simulink model "SF044A_HowDetn"  (R2013b)
settings: Solver=FixedStepDiscrete  SolverMode=SingleTasking  StartTime=0.0  StopTime=1  FixedStep=0.002  RelTol=1e-3
values from neighbouring files (symbols this model uses):
  ABSLTHIFRQTQHILIM_HWNWTMTR_F32 = DataDict.Constant    [SF044A_HowDetn_DataDict.m]
  ABSLTHIFRQTQLOLIM_HWNWTMTR_F32 = DataDict.Constant    [SF044A_HowDetn_DataDict.m]
  ARCHGLBPRM_2MILLISEC_SEC_F32 = DataDict.Constant    [SF044A_HowDetn_DataDict.m]
  HOWDETNESTIMNLIM_ULS_F32 = DataDict.Constant    [SF044A_HowDetn_DataDict.m]
  HOWDETNESTIMNTHD_ULS_F32 = DataDict.Constant    [SF044A_HowDetn_DataDict.m]
  HowDetnHiFrqGainY = DataDict.Calibration    [SF044A_HowDetn_DataDict.m]
  HowDetnMinVehSpd = DataDict.Calibration    [SF044A_HowDetn_DataDict.m]
  HowDetnOffThd = DataDict.Calibration    [SF044A_HowDetn_DataDict.m]
  HowDetnOffTi = DataDict.Calibration    [SF044A_HowDetn_DataDict.m]
  HowDetnPercOfPrevHowEstim = DataDict.Calibration    [SF044A_HowDetn_DataDict.m]
  HowDetnSlewRate = DataDict.Calibration    [SF044A_HowDetn_DataDict.m]
  HowDetnVehSpd = DataDict.Calibration    [SF044A_HowDetn_DataDict.m]
  HUNDREDMICROSECTOMILLISEC_ULS_F32 = DataDict.Constant    [SF044A_HowDetn_DataDict.m]
  MILLISECTOSEC_ULS_F32 = DataDict.Constant    [SF044A_HowDetn_DataDict.m]
libraries: Fil x14, FloatToFixd x6, NxtrLim x5, FixdToFloat x4, BilnrIntrpnMplX x2, NxtrAbslt x2, simulink x2, LnrIntrpn x1, LnrIntrpnDyn x1
(part 2 of 2)

== system SF044A_HowDetn/HowDetn/HowDetnPer1/Calculate HOW Estimate/Low-Frequency Lookup Table ==
  VehSpd : Inport
  AbsLoFrqTq : Inport  Port=2
  BilnrIntrpnWithRound_s16_u16MplXs16MplY : BilnrIntrpnMplX/BilnrIntrpnWithRound_s16_u16MplXs16MplY  MplXTbl=HowDetnLoFrqRateX  MplYTbl=HowDetnLoFrqRateY  BilnrSelnTbl=HowDetnVehSpd
      settings: AttributesFormatString=Bilnr ( u16MplX , s16MplY )
  CopyRight2 : Subsystem  Description=|  mask(Copyright Information){none=on}
      | Copyright info block.                                               
      |                                                                     
      | Place copyright information at the top of every subsystem in design.
      mask prompts: none "No parameters"
      mask help: Place copyright information at the top of every subsystem in design.
      mask Display:
      | NxtrConf = 'Nexteer Confidential';
      | 
      | sys = bdroot; %handle for the current model ("system")
      | first = get_param(sys,'Created');
      | first = first(end-3:end);  %year is last four digits
      | 
      | last = get_param(sys,'LastModifiedDate');
      | if isempty(last)
      |     last = datestr(now,'yyyy');
      | else
      |     last = last(end-3:end);
      | end
      | 
      | if strcmp(first,last)
      |     fprintf('%s -- Copyright %s Nexteer',NxtrConf,first)
      | else
      |     fprintf('%s -- %s%s- %s Nexteer',NxtrConf,char(169),first,last)
      | end
  FixdToFloat_f32_s16 : FixdToFloat/FixdToFloat_f32_s16  Param1=8
  FloatToFixd_u16_f1 : FloatToFixd/FloatToFixd_u16_f32  Param1=8
  FloatToFixd_u16_f32 : FloatToFixd/FloatToFixd_u16_f32  Param1=7
  LoFrqRateY : Outport
  wires:
  FloatToFixd_u16_f32/1 -> BilnrIntrpnWithRound_s16_u16MplXs16MplY/2
  BilnrIntrpnWithRound_s16_u16MplXs16MplY/1 -> FixdToFloat_f32_s16/1
  FloatToFixd_u16_f1/1 -> BilnrIntrpnWithRound_s16_u16MplXs16MplY/1
  VehSpd/1 -> FloatToFixd_u16_f32/1
  AbsLoFrqTq/1 -> FloatToFixd_u16_f1/1
  FixdToFloat_f32_s16/1 -> LoFrqRateY/1

== system SF044A_HowDetn/HowDetn/HowDetnPer1/Calculate HOW Estimate/default ==
  Action Port : ActionPort  ActionType=else
  Constant : Constant  RequirementInfo={} %GIDa_67017ff9_6322_4976_b2c8_c00694960ef8  Value=HOWDETNESTIMNTHD_ULS_F32  OutDataTypeStr=single
  CopyRight2 : Subsystem  Description=|  mask(Copyright Information){none=on}
      | Copyright info block.                                               
      |                                                                     
      | Place copyright information at the top of every subsystem in design.
      mask prompts: none "No parameters"
      mask help: Place copyright information at the top of every subsystem in design.
      mask Display:
      | NxtrConf = 'Nexteer Confidential';
      | 
      | sys = bdroot; %handle for the current model ("system")
      | first = get_param(sys,'Created');
      | first = first(end-3:end);  %year is last four digits
      | 
      | last = get_param(sys,'LastModifiedDate');
      | if isempty(last)
      |     last = datestr(now,'yyyy');
      | else
      |     last = last(end-3:end);
      | end
      | 
      | if strcmp(first,last)
      |     fprintf('%s -- Copyright %s Nexteer',NxtrConf,first)
      | else
      |     fprintf('%s -- %s%s- %s Nexteer',NxtrConf,char(169),first,last)
      | end
  Out : Outport
  wires:
  Constant/1 -> Out/1

== system SF044A_HowDetn/HowDetn/HowDetnPer1/Determine HOW Flag/CopyRight2 ==

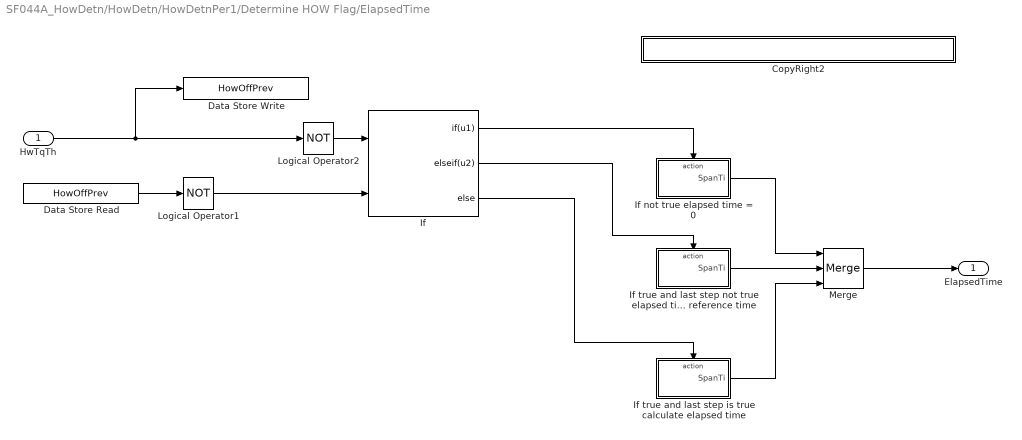
== system SF044A_HowDetn/HowDetn/HowDetnPer1/Determine HOW Flag/ElapsedTime ==
  HwTqTh : Inport
  CopyRight2 : Subsystem  Description=|  mask(Copyright Information){none=on}
      | Copyright info block.                                               
      |                                                                     
      | Place copyright information at the top of every subsystem in design.
      mask prompts: none "No parameters"
      mask help: Place copyright information at the top of every subsystem in design.
      mask Display:
      | NxtrConf = 'Nexteer Confidential';
      | 
      | sys = bdroot; %handle for the current model ("system")
      | first = get_param(sys,'Created');
      | first = first(end-3:end);  %year is last four digits
      | 
      | last = get_param(sys,'LastModifiedDate');
      | if isempty(last)
      |     last = datestr(now,'yyyy');
      | else
      |     last = last(end-3:end);
      | end
      | 
      | if strcmp(first,last)
      |     fprintf('%s -- Copyright %s Nexteer',NxtrConf,first)
      | else
      |     fprintf('%s -- %s%s- %s Nexteer',NxtrConf,char(169),first,last)
      | end
  Data Store Read : DataStoreRead  Priority=0  DataStoreName=HowOffPrev
      settings: AttributesFormatString=Priority: %<Priority>
  Data Store Write : DataStoreWrite  Priority=1  DataStoreName=HowOffPrev
      settings: AttributesFormatString=Priority: %<Priority>
  If : If  NumInputs=2  IfExpression=u1  ElseIfExpressions=u2
  If not true elapsed time = 0 : Subsystem  TreatAsAtomicUnit=on
  "If true and last step is true calculate elapsed time " : Subsystem  TreatAsAtomicUnit=on
  "If true and last step not true elapsed time = 0 get reference time " : Subsystem  TreatAsAtomicUnit=on
  Logical Operator1 : Logic  Operator=NOT  AllPortsSameDT=off  OutDataTypeStr=boolean
  Logical Operator2 : Logic  Operator=NOT  AllPortsSameDT=off  OutDataTypeStr=boolean
  Merge : Merge  Inputs=3
  ElapsedTime : Outport
  wires:
  If/1 -> If not true elapsed time = 0/Action
  If/2 -> "If true and last step not true elapsed time = 0 get reference time "/Action
  If/3 -> "If true and last step is true calculate elapsed time "/Action
  If not true elapsed time = 0/1(SpanTi) -> Merge/1
  "If true and last step not true elapsed time = 0 get reference time "/1("SpanTi ") -> Merge/2
  "If true and last step is true calculate elapsed time "/1(SpanTi) -> Merge/3
  Merge/1 -> ElapsedTime/1
  HwTqTh/1 -> Logical Operator2/1, Data Store Write/1
  Data Store Read/1 -> Logical Operator1/1
  Logical Operator2/1 -> If/1
  Logical Operator1/1 -> If/2

== system SF044A_HowDetn/HowDetn/HowDetnPer1/Determine HOW Flag/HandsOffDetn ==
  Action Port : ActionPort  ActionType=then
  CopyRight2 : Subsystem  Description=|  mask(Copyright Information){none=on}
      | Copyright info block.                                               
      |                                                                     
      | Place copyright information at the top of every subsystem in design.
      mask prompts: none "No parameters"
      mask help: Place copyright information at the top of every subsystem in design.
      mask Display:
      | NxtrConf = 'Nexteer Confidential';
      | 
      | sys = bdroot; %handle for the current model ("system")
      | first = get_param(sys,'Created');
      | first = first(end-3:end);  %year is last four digits
      | 
      | last = get_param(sys,'LastModifiedDate');
      | if isempty(last)
      |     last = datestr(now,'yyyy');
      | else
      |     last = last(end-3:end);
      | end
      | 
      | if strcmp(first,last)
      |     fprintf('%s -- Copyright %s Nexteer',NxtrConf,first)
      | else
      |     fprintf('%s -- %s%s- %s Nexteer',NxtrConf,char(169),first,last)
      | end
  Hands Off Wheel : Constant  RequirementInfo={} %GIDa_d4e6488b_e252_4824_9c02_dd6a1a50822f  Value=false  OutDataTypeStr=boolean
  HowDetnFlg : Outport
  wires:
  Hands Off Wheel/1 -> HowDetnFlg/1

== system SF044A_HowDetn/HowDetn/HowDetnPer1/Determine HOW Flag/HandsOnDetn ==
  Action Port : ActionPort  ActionType=else
  CopyRight2 : Subsystem  Description=|  mask(Copyright Information){none=on}
      | Copyright info block.                                               
      |                                                                     
      | Place copyright information at the top of every subsystem in design.
      mask prompts: none "No parameters"
      mask help: Place copyright information at the top of every subsystem in design.
      mask Display:
      | NxtrConf = 'Nexteer Confidential';
      | 
      | sys = bdroot; %handle for the current model ("system")
      | first = get_param(sys,'Created');
      | first = first(end-3:end);  %year is last four digits
      | 
      | last = get_param(sys,'LastModifiedDate');
      | if isempty(last)
      |     last = datestr(now,'yyyy');
      | else
      |     last = last(end-3:end);
      | end
      | 
      | if strcmp(first,last)
      |     fprintf('%s -- Copyright %s Nexteer',NxtrConf,first)
      | else
      |     fprintf('%s -- %s%s- %s Nexteer',NxtrConf,char(169),first,last)
      | end
  Hands On Wheel : Constant  RequirementInfo={} %GIDa_8392a09a_cc4f_428e_9a0f_d9eb35861263  Value=true  OutDataTypeStr=boolean
  HowDetnFlg : Outport
  wires:
  Hands On Wheel/1 -> HowDetnFlg/1

== system SF044A_HowDetn/HowDetn/HowDetnPer1/Determine HOW State/CopyRight2 ==

== system SF044A_HowDetn/HowDetn/HowDetnPer1/Determine HOW State/HOW State Look up Table ==
  HowEstimFil : Inport
  CopyRight2 : Subsystem  Description=|  mask(Copyright Information){none=on}
      | Copyright info block.                                               
      |                                                                     
      | Place copyright information at the top of every subsystem in design.
      mask prompts: none "No parameters"
      mask help: Place copyright information at the top of every subsystem in design.
      mask Display:
      | NxtrConf = 'Nexteer Confidential';
      | 
      | sys = bdroot; %handle for the current model ("system")
      | first = get_param(sys,'Created');
      | first = first(end-3:end);  %year is last four digits
      | 
      | last = get_param(sys,'LastModifiedDate');
      | if isempty(last)
      |     last = datestr(now,'yyyy');
      | else
      |     last = last(end-3:end);
      | end
      | 
      | if strcmp(first,last)
      |     fprintf('%s -- Copyright %s Nexteer',NxtrConf,first)
      | else
      |     fprintf('%s -- %s%s- %s Nexteer',NxtrConf,char(169),first,last)
      | end
  Data Type Conversion : DataTypeConversion  OutDataTypeStr=int8
  FloatToFixd_u16_f1 : FloatToFixd/FloatToFixd_u16_f32  Param1=8
  LnrIntrpn_s16_u16VariXs16VariY : LnrIntrpn/LnrIntrpn_s16_u16VariXs16VariY  RequirementInfo={} %GIDa_1ceff8d9_cb44_435a_8fb8_bb742ada6bbe  XTbl=HowDetnStThdX  YTbl=HOWSTY_CNT_S15P0
      settings: AttributesFormatString=Lnr ( u16VariX , s16VariY )
  HowDetnSt : Outport
  wires:
  HowEstimFil/1 -> FloatToFixd_u16_f1/1
  FloatToFixd_u16_f1/1 -> LnrIntrpn_s16_u16VariXs16VariY/1
  LnrIntrpn_s16_u16VariXs16VariY/1 -> Data Type Conversion/1
  Data Type Conversion/1 -> HowDetnSt/1

== system SF044A_HowDetn/HowDetn/HowDetnPer1/Determine HOW State/Pass ==
  Input : Inport
  Action Port : ActionPort  ActionType=then
  CopyRight2 : Subsystem  Description=|  mask(Copyright Information){none=on}
      | Copyright info block.                                               
      |                                                                     
      | Place copyright information at the top of every subsystem in design.
      mask prompts: none "No parameters"
      mask help: Place copyright information at the top of every subsystem in design.
      mask Display:
      | NxtrConf = 'Nexteer Confidential';
      | 
      | sys = bdroot; %handle for the current model ("system")
      | first = get_param(sys,'Created');
      | first = first(end-3:end);  %year is last four digits
      | 
      | last = get_param(sys,'LastModifiedDate');
      | if isempty(last)
      |     last = datestr(now,'yyyy');
      | else
      |     last = last(end-3:end);
      | end
      | 
      | if strcmp(first,last)
      |     fprintf('%s -- Copyright %s Nexteer',NxtrConf,first)
      | else
      |     fprintf('%s -- %s%s- %s Nexteer',NxtrConf,char(169),first,last)
      | end
  HowDetnSt : Outport
  wires:
  Input/1 -> HowDetnSt/1

== system SF044A_HowDetn/HowDetn/HowDetnPer1/Determine HOW State/Zero ==
  Action Port : ActionPort  ActionType=else
  Constant : Constant  Value=0  OutDataTypeStr=int8
      settings: AttributesFormatString=%<OutDataTypeStr>
  CopyRight2 : Subsystem  Description=|  mask(Copyright Information){none=on}
      | Copyright info block.                                               
      |                                                                     
      | Place copyright information at the top of every subsystem in design.
      mask prompts: none "No parameters"
      mask help: Place copyright information at the top of every subsystem in design.
      mask Display:
      | NxtrConf = 'Nexteer Confidential';
      | 
      | sys = bdroot; %handle for the current model ("system")
      | first = get_param(sys,'Created');
      | first = first(end-3:end);  %year is last four digits
      | 
      | last = get_param(sys,'LastModifiedDate');
      | if isempty(last)
      |     last = datestr(now,'yyyy');
      | else
      |     last = last(end-3:end);
      | end
      | 
      | if strcmp(first,last)
      |     fprintf('%s -- Copyright %s Nexteer',NxtrConf,first)
      | else
      |     fprintf('%s -- %s%s- %s Nexteer',NxtrConf,char(169),first,last)
      | end
  HowDetnSt : Outport
  wires:
  Constant/1 -> HowDetnSt/1

== system SF044A_HowDetn/HowDetn/HowDetnPer1/Filter HwTq/CopyRight2 ==

== system SF044A_HowDetn/HowDetn/HowDetnPer1/Calculate HOW Estimate/CalcEstimn/CopyRight2 ==

== system SF044A_HowDetn/HowDetn/HowDetnPer1/Calculate HOW Estimate/High-Frequency Lookup Table/CopyRight2 ==

== system SF044A_HowDetn/HowDetn/HowDetnPer1/Calculate HOW Estimate/Low-Frequency Lookup Table/CopyRight2 ==

== system SF044A_HowDetn/HowDetn/HowDetnPer1/Calculate HOW Estimate/default/CopyRight2 ==

== system SF044A_HowDetn/HowDetn/HowDetnPer1/Determine HOW Flag/ElapsedTime/CopyRight2 ==

== system SF044A_HowDetn/HowDetn/HowDetnPer1/Determine HOW Flag/ElapsedTime/If not true elapsed time = 0 ==
  Action Port : ActionPort  ActionType=then
  Constant : Constant  Value=0  OutDataTypeStr=single
  CopyRight2 : Subsystem  Description=|  mask(Copyright Information){none=on}
      | Copyright info block.                                               
      |                                                                     
      | Place copyright information at the top of every subsystem in design.
      mask prompts: none "No parameters"
      mask help: Place copyright information at the top of every subsystem in design.
      mask Display:
      | NxtrConf = 'Nexteer Confidential';
      | 
      | sys = bdroot; %handle for the current model ("system")
      | first = get_param(sys,'Created');
      | first = first(end-3:end);  %year is last four digits
      | 
      | last = get_param(sys,'LastModifiedDate');
      | if isempty(last)
      |     last = datestr(now,'yyyy');
      | else
      |     last = last(end-3:end);
      | end
      | 
      | if strcmp(first,last)
      |     fprintf('%s -- Copyright %s Nexteer',NxtrConf,first)
      | else
      |     fprintf('%s -- %s%s- %s Nexteer',NxtrConf,char(169),first,last)
      | end
  SpanTi : Outport
  wires:
  Constant/1 -> SpanTi/1

== system SF044A_HowDetn/HowDetn/HowDetnPer1/Determine HOW Flag/ElapsedTime/If true and last step is true calculate elapsed time  ==
  Action Port : ActionPort  ActionType=else
  Constant1 : Constant  Value=HUNDREDMICROSECTOMILLISEC_ULS_F32
  CopyRight2 : Subsystem  Description=|  mask(Copyright Information){none=on}
      | Copyright info block.                                               
      |                                                                     
      | Place copyright information at the top of every subsystem in design.
      mask prompts: none "No parameters"
      mask help: Place copyright information at the top of every subsystem in design.
      mask Display:
      | NxtrConf = 'Nexteer Confidential';
      | 
      | sys = bdroot; %handle for the current model ("system")
      | first = get_param(sys,'Created');
      | first = first(end-3:end);  %year is last four digits
      | 
      | last = get_param(sys,'LastModifiedDate');
      | if isempty(last)
      |     last = datestr(now,'yyyy');
      | else
      |     last = last(end-3:end);
      | end
      | 
      | if strcmp(first,last)
      |     fprintf('%s -- Copyright %s Nexteer',NxtrConf,first)
      | else
      |     fprintf('%s -- %s%s- %s Nexteer',NxtrConf,char(169),first,last)
      | end
  Data Store Read : DataStoreRead  DataStoreName=RefTiHowOff
  Divide : Product  Inputs=**
  FixdToFloat_f32_u32 : FixdToFloat/FixdToFloat_f32_u32  Param1=0
  GetTiSpan100MicroSec32bit : Subsystem  mask(Timer_GTS){}
      mask help: Used to get the time span between start and current time.
  SpanTi : Outport
  wires:
  Divide/1 -> SpanTi/1
  GetTiSpan100MicroSec32bit/1(TiSpan) -> FixdToFloat_f32_u32/1
  Data Store Read/1 -> GetTiSpan100MicroSec32bit/1(RefTmr)
  FixdToFloat_f32_u32/1 -> Divide/1
  Constant1/1 -> Divide/2

== system SF044A_HowDetn/HowDetn/HowDetnPer1/Determine HOW Flag/ElapsedTime/If true and last step not true elapsed time = 0 get reference time  ==
  Action Port : ActionPort  ActionType=elseif
  Constant : Constant  Value=0  OutDataTypeStr=single
  CopyRight2 : Subsystem  Description=|  mask(Copyright Information){none=on}
      | Copyright info block.                                               
      |                                                                     
      | Place copyright information at the top of every subsystem in design.
      mask prompts: none "No parameters"
      mask help: Place copyright information at the top of every subsystem in design.
      mask Display:
      | NxtrConf = 'Nexteer Confidential';
      | 
      | sys = bdroot; %handle for the current model ("system")
      | first = get_param(sys,'Created');
      | first = first(end-3:end);  %year is last four digits
      | 
      | last = get_param(sys,'LastModifiedDate');
      | if isempty(last)
      |     last = datestr(now,'yyyy');
      | else
      |     last = last(end-3:end);
      | end
      | 
      | if strcmp(first,last)
      |     fprintf('%s -- Copyright %s Nexteer',NxtrConf,first)
      | else
      |     fprintf('%s -- %s%s- %s Nexteer',NxtrConf,char(169),first,last)
      | end
  Data Store Write : DataStoreWrite  DataStoreName=RefTiHowOff
  GetRefTmr100MicroSec32bit1 : Subsystem  mask(Timer_GRF){}
      mask help: Used to get the reference time in a model.
  "SpanTi " : Outport
  wires:
  Constant/1 -> "SpanTi "/1
  GetRefTmr100MicroSec32bit1/1(RefTmr) -> Data Store Write/1

== system SF044A_HowDetn/HowDetn/HowDetnPer1/Determine HOW Flag/HandsOffDetn/CopyRight2 ==

== system SF044A_HowDetn/HowDetn/HowDetnPer1/Determine HOW Flag/HandsOnDetn/CopyRight2 ==

== system SF044A_HowDetn/HowDetn/HowDetnPer1/Determine HOW State/HOW State Look up Table/CopyRight2 ==

== system SF044A_HowDetn/HowDetn/HowDetnPer1/Determine HOW State/Pass/CopyRight2 ==

== system SF044A_HowDetn/HowDetn/HowDetnPer1/Determine HOW State/Zero/CopyRight2 ==

== system SF044A_HowDetn/HowDetn/HowDetnPer1/Determine HOW Flag/ElapsedTime/If not true elapsed time = 0/CopyRight2 ==

== system SF044A_HowDetn/HowDetn/HowDetnPer1/Determine HOW Flag/ElapsedTime/If true and last step is true calculate elapsed time /CopyRight2 ==

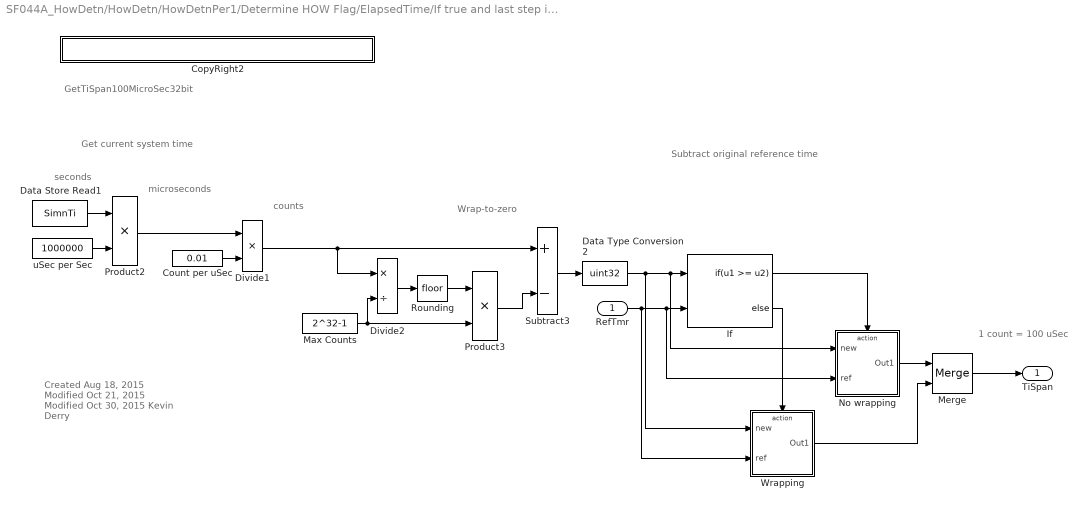
== system SF044A_HowDetn/HowDetn/HowDetnPer1/Determine HOW Flag/ElapsedTime/If true and last step is true calculate elapsed time /GetTiSpan100MicroSec32bit ==
  note: Subtract original reference time
  note: seconds
  note: microseconds
  note: counts
  note: Wrap-to-zero
  note: 1 count = 100 uSec
  note: Get current system time
  note: GetTiSpan100MicroSec32bit
  note: Created Aug 18, 2015
      | Modified Oct 21, 2015
      | Modified Oct 30, 2015
      | Kevin Derry
  RefTmr : Inport
  CopyRight2 : Subsystem  Description=|  mask(Copyright Information){none=on}
      | Copyright info block.                                               
      |                                                                     
      | Place copyright information at the top of every subsystem in design.
      mask prompts: none "No parameters"
      mask help: Place copyright information at the top of every subsystem in design.
      mask Display:
      | NxtrConf = 'Nexteer Confidential';
      | 
      | sys = bdroot; %handle for the current model ("system")
      | first = get_param(sys,'Created');
      | if(isempty(first))
      |     first = datestr(now,'yyyy');
      | else
      |     first = first(end-3:end);  %year is last four digits
      | end
      | 
      | last = get_param(sys,'LastModifiedDate');
      | if isempty(last)
      |     last = datestr(now,'yyyy');
      | else
      |     last = last(end-3:end);
      | end
      | 
      | if strcmp(first,last)
      |     fprintf('%s -- Copyright %s Nexteer',NxtrConf,first)
      | else
      |     fprintf('%s -- %s%s- %s Nexteer',NxtrConf,char(169),first,last)
      | end
  Count per uSec : Constant  Value=0.01
  Data Store Read1 : DataStoreRead  DataStoreName=SimnTi
  Data Type Conversion2 : DataTypeConversion  OutDataTypeStr=uint32
  Divide1 : Product  Inputs=**
  Divide2 : Product  Inputs=*/
  If : If  NumInputs=2  IfExpression=u1 >= u2
  Max Counts : Constant  Value=2^32-1
  Merge : Merge
  No wrapping : Subsystem  TreatAsAtomicUnit=on
  Product2 : Product
  Product3 : Product
  Rounding : Rounding
  Subtract3 : Sum  Inputs=+-
  Wrapping : Subsystem  TreatAsAtomicUnit=on
  uSec per Sec : Constant  Value=1000000
  TiSpan : Outport
  wires:
  Wrapping/1(Out1) -> Merge/2
  No wrapping/1(Out1) -> Merge/1
  If/2 -> Wrapping/Action
  If/1 -> No wrapping/Action
  Product3/1 -> Subtract3/2
  Subtract3/1 -> Data Type Conversion2/1
  Rounding/1 -> Product3/1
  Divide2/1 -> Rounding/1
  Max Counts/1 -> Divide2/2, Product3/2
  Divide1/1 -> Divide2/1, Subtract3/1
  Product2/1 -> Divide1/1
  Data Store Read1/1 -> Product2/1
  Count per uSec/1 -> Divide1/2
  uSec per Sec/1 -> Product2/2
  Merge/1 -> TiSpan/1
  RefTmr/1 -> If/2, No wrapping/2(ref), Wrapping/2(ref)
  Data Type Conversion2/1 -> If/1, No wrapping/1(new), Wrapping/1(new)

== system SF044A_HowDetn/HowDetn/HowDetnPer1/Determine HOW Flag/ElapsedTime/If true and last step not true elapsed time = 0 get reference time /CopyRight2 ==

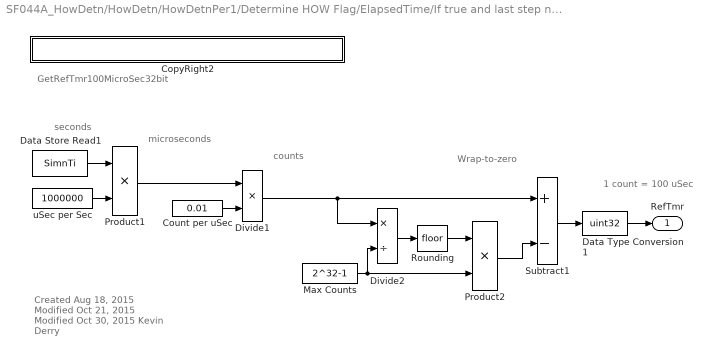
== system SF044A_HowDetn/HowDetn/HowDetnPer1/Determine HOW Flag/ElapsedTime/If true and last step not true elapsed time = 0 get reference time /GetRefTmr100MicroSec32bit1 ==
  note: 1 count = 100 uSec
  note: seconds
  note: microseconds
  note: counts
  note: Wrap-to-zero
  note: GetRefTmr100MicroSec32bit
  note: Created Aug 18, 2015
      | Modified Oct 21, 2015
      | Modified Oct 30, 2015
      | Kevin Derry
  CopyRight2 : Subsystem  Description=|  mask(Copyright Information){none=on}
      | Copyright info block.                                               
      |                                                                     
      | Place copyright information at the top of every subsystem in design.
      mask prompts: none "No parameters"
      mask help: Place copyright information at the top of every subsystem in design.
      mask Display:
      | NxtrConf = 'Nexteer Confidential';
      | 
      | sys = bdroot; %handle for the current model ("system")
      | first = get_param(sys,'Created');
      | if(isempty(first))
      |     first = datestr(now,'yyyy');
      | else
      |     first = first(end-3:end);  %year is last four digits
      | end
      | 
      | last = get_param(sys,'LastModifiedDate');
      | if isempty(last)
      |     last = datestr(now,'yyyy');
      | else
      |     last = last(end-3:end);
      | end
      | 
      | if strcmp(first,last)
      |     fprintf('%s -- Copyright %s Nexteer',NxtrConf,first)
      | else
      |     fprintf('%s -- %s%s- %s Nexteer',NxtrConf,char(169),first,last)
      | end
  Count per uSec : Constant  Value=0.01
  Data Store Read1 : DataStoreRead  DataStoreName=SimnTi
  Data Type Conversion1 : DataTypeConversion  OutDataTypeStr=uint32
  Divide1 : Product  Inputs=**
  Divide2 : Product  Inputs=*/
  Max Counts : Constant  Value=2^32-1
  Product1 : Product
  Product2 : Product
  Rounding : Rounding
  Subtract1 : Sum  Inputs=+-
  uSec per Sec : Constant  Value=1000000
  RefTmr : Outport
  wires:
  Product2/1 -> Subtract1/2
  Subtract1/1 -> Data Type Conversion1/1
  Rounding/1 -> Product2/1
  Divide2/1 -> Rounding/1
  Max Counts/1 -> Divide2/2, Product2/2
  Divide1/1 -> Divide2/1, Subtract1/1
  Product1/1 -> Divide1/1
  Count per uSec/1 -> Divide1/2
  uSec per Sec/1 -> Product1/2
  Data Type Conversion1/1 -> RefTmr/1
  Data Store Read1/1 -> Product1/1

== system SF044A_HowDetn/HowDetn/HowDetnPer1/Determine HOW Flag/ElapsedTime/If true and last step is true calculate elapsed time /GetTiSpan100MicroSec32bit/CopyRight2 ==

== system SF044A_HowDetn/HowDetn/HowDetnPer1/Determine HOW Flag/ElapsedTime/If true and last step is true calculate elapsed time /GetTiSpan100MicroSec32bit/No wrapping ==
  new : Inport
  ref : Inport  Port=2
  Action Port : ActionPort  ActionType=then
  CopyRight2 : Subsystem  Description=|  mask(Copyright Information){none=on}
      | Copyright info block.                                               
      |                                                                     
      | Place copyright information at the top of every subsystem in design.
      mask prompts: none "No parameters"
      mask help: Place copyright information at the top of every subsystem in design.
      mask Display:
      | NxtrConf = 'Nexteer Confidential';
      | 
      | sys = bdroot; %handle for the current model ("system")
      | first = get_param(sys,'Created');
      | if(isempty(first))
      |     first = datestr(now,'yyyy');
      | else
      |     first = first(end-3:end);  %year is last four digits
      | end
      | 
      | last = get_param(sys,'LastModifiedDate');
      | if isempty(last)
      |     last = datestr(now,'yyyy');
      | else
      |     last = last(end-3:end);
      | end
      | 
      | if strcmp(first,last)
      |     fprintf('%s -- Copyright %s Nexteer',NxtrConf,first)
      | else
      |     fprintf('%s -- %s%s- %s Nexteer',NxtrConf,char(169),first,last)
      | end
  Subtract1 : Sum  Inputs=+-
  Out1 : Outport
  wires:
  ref/1 -> Subtract1/2
  new/1 -> Subtract1/1
  Subtract1/1 -> Out1/1

== system SF044A_HowDetn/HowDetn/HowDetnPer1/Determine HOW Flag/ElapsedTime/If true and last step is true calculate elapsed time /GetTiSpan100MicroSec32bit/Wrapping ==
  new : Inport
  ref : Inport  Port=2
  Action Port : ActionPort  ActionType=else
  CopyRight2 : Subsystem  Description=|  mask(Copyright Information){none=on}
      | Copyright info block.                                               
      |                                                                     
      | Place copyright information at the top of every subsystem in design.
      mask prompts: none "No parameters"
      mask help: Place copyright information at the top of every subsystem in design.
      mask Display:
      | NxtrConf = 'Nexteer Confidential';
      | 
      | sys = bdroot; %handle for the current model ("system")
      | first = get_param(sys,'Created');
      | if(isempty(first))
      |     first = datestr(now,'yyyy');
      | else
      |     first = first(end-3:end);  %year is last four digits
      | end
      | 
      | last = get_param(sys,'LastModifiedDate');
      | if isempty(last)
      |     last = datestr(now,'yyyy');
      | else
      |     last = last(end-3:end);
      | end
      | 
      | if strcmp(first,last)
      |     fprintf('%s -- Copyright %s Nexteer',NxtrConf,first)
      | else
      |     fprintf('%s -- %s%s- %s Nexteer',NxtrConf,char(169),first,last)
      | end
  Max Counts : Constant  Value=2^32-1  OutDataTypeStr=uint32
  Subtract1 : Sum  Inputs=+-+
  Out1 : Outport
  wires:
  new/1 -> Subtract1/3
  ref/1 -> Subtract1/2
  Max Counts/1 -> Subtract1/1
  Subtract1/1 -> Out1/1

== system SF044A_HowDetn/HowDetn/HowDetnPer1/Determine HOW Flag/ElapsedTime/If true and last step not true elapsed time = 0 get reference time /GetRefTmr100MicroSec32bit1/CopyRight2 ==

== system SF044A_HowDetn/HowDetn/HowDetnPer1/Determine HOW Flag/ElapsedTime/If true and last step is true calculate elapsed time /GetTiSpan100MicroSec32bit/No wrapping/CopyRight2 ==

== system SF044A_HowDetn/HowDetn/HowDetnPer1/Determine HOW Flag/ElapsedTime/If true and last step is true calculate elapsed time /GetTiSpan100MicroSec32bit/Wrapping/CopyRight2 ==
